simulink model "tf_vary"  (R2020a)
settings: Solver=ode45  StartTime=0.0  StopTime=10.0  FixedStep=0.001  RelTol=1e-3
values from neighbouring files (symbols this model uses):
  Kd = 3.2058    [ModifiedFitness.m]    (also in PSO_Optim.m = x(3); itae_cost.m = x(3); main_ga.m = x(3); pid_optim.m = x(3))
  Ki = 7.7194e+03    (= 7719.4)    [ModifiedFitness.m]    (also in PSO_Optim.m = x(2); itae_cost.m = x(2); main_ga.m = x(2); pid_optim.m = x(2))
  Kp = 305.4814    [ModifiedFitness.m]    (also in PSO_Optim.m = x(1); itae_cost.m = x(1); main_ga.m = x(1); pid_optim.m = x(1))
settings Model: Creator=vic  LastModifiedBy=Mitterrand Ekole
settings DataIOCC: ReturnWorkspaceOutputs=off
settings DebuggingCC: ArithmeticOperatorsInVariantConditions=warning
settings SFSimCC: SimUseLocalCustomCode=off  CustomCodeUndefinedFunction=UseInterfaceOnly
settings RTWCC: RTWUseLocalCustomCode=off

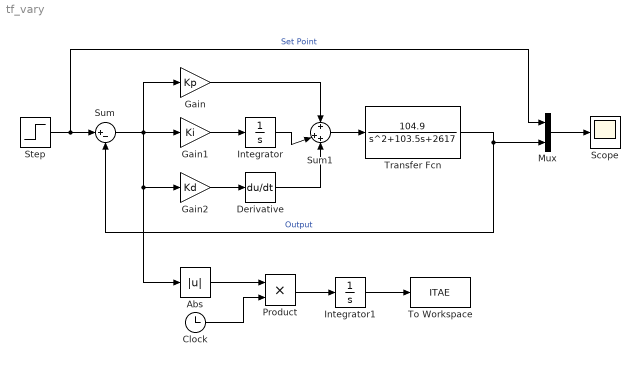
== system tf_vary ==
  Abs : Abs
  Clock : Clock
  Derivative : Derivative
  Gain : Gain  Gain=Kp
  Gain1 : Gain  Gain=Ki
  Gain2 : Gain  Gain=Kd
  Integrator : Integrator
  Integrator1 : Integrator
  Mux : Mux  Inputs=2
  Product : Product
  Scope : Scope
  Step : Step  Time=0  SampleTime=0
  Sum : Sum  Inputs=|+-
  Sum1 : Sum  Inputs=+|++
  To Workspace : ToWorkspace  VariableName=ITAE  SampleTime=-1
  Transfer Fcn : TransferFcn  Numerator=[104.9]  Denominator=[1 103.5 2617]
  wires:
  Transfer Fcn/1 -> Mux/2, Sum/2  "Output"
  Step/1 -> Mux/1, Sum/1  "Set Point"
  Sum1/1 -> Transfer Fcn/1
  Gain1/1 -> Integrator/1
  Gain2/1 -> Derivative/1
  Integrator/1 -> Sum1/2
  Gain/1 -> Sum1/1
  Derivative/1 -> Sum1/3
  Sum/1 -> Abs/1, Gain2/1, Gain/1, Gain1/1
  Mux/1 -> Scope/1
  Abs/1 -> Product/1
  Clock/1 -> Product/2
  Product/1 -> Integrator1/1
  Integrator1/1 -> To Workspace/1
